simulink model "WithLoad_Simple"  (R2017b)
settings: Solver=ode3  StartTime=0.0  StopTime=10  FixedStep=0.005  RelTol=1e-3  EnableMultiTasking=on
libraries: mblibv1 x61
(part 1 of 3)
settings Model: MAModelExclusionFileProxy=C:\Users\Jiao\Documents\MATLAB\ARNSC_identify_DYN_para\WithLoad_Simple_exclusions.xml  Creator=Robot_One  LastModifiedBy=Chunting
settings DataIOCC: LimitDataPoints=on  SaveFormat=Array
settings OptimizationCC: ExpressionDepthLimit=2147483647  LifeSpan=inf
settings DebuggingCC: UnderspecifiedInitializationDetection=Classic  MergeDetectMultiDrivingBlocksExec=none  SolverPrmCheckMsg=warning  StateNameClashWarn=warning  SFUnexpectedBacktrackingDiag=warning  SFNoUnconditionalDefaultTransitionDiag=warning  SFExecutionAtInitializationDiag=none
settings HardwareCC: ProdBitPerPointer=32  ProdBitPerSizeT=32  ProdBitPerPtrDiffT=32  ProdLargestAtomicFloat=None  ProdIntDivRoundTo=Undefined  ProdEndianess=Unspecified  ProdWordSize=32  ProdHWDeviceType=32-bit Generic
settings ModelReferenceCC: PropagateSignalLabelsOutOfModel=off
settings CodeAppCC: StateflowObjectComments=on
settings GRTTargetCC: TargetLangStandard=C89/C90 (ANSI)  GeneratePreprocessorConditionals=Disable all
settings ConfigComp: CovMetricSettings=dw  CovHtmlReporting=on  CovSaveCumulativeToWorkspaceVar=on  CovSaveSingleToWorkspaceVar=on  CovExternalEMLEnable=off
settings SimscapeCC: SimscapeNormalizeSystem=off
settings SimMechanicsCC: VisDuringSimulation=on  HighlightModel=off  AutoFitVis=GROWTOFIT  LastVizWinPosition=[1 41 1366 626]  CamPosition=[-3.72812;3.39912;13.5529;]  CamTarget=[1.16146;-0.0373873;0.128842;]  CamUpVector=[0.163931;0.968356;-0.188185;]  CamHeight=2.35418  VisBackgroundColor=[0;0;0;]  DefaultBodyColor=[1;0;0;]
settings ConfigurationSet: Description=SimMechanics 2G

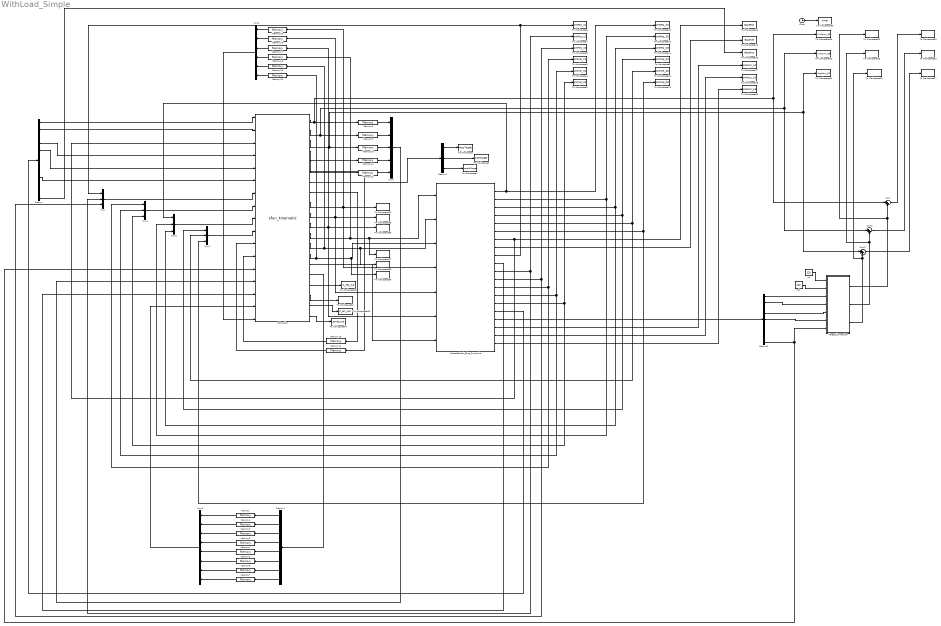
== system WithLoad_Simple ==
  Clock : Clock
  Demux : Demux  Outputs=12
  Demux1 : Demux  Outputs=8
  Demux2 : Demux  Outputs=9
  Demux4 : Demux  Outputs=3
  Memory{,1..10,12..20} (20 alike) : Memory
  Memory11 : Memory  InitialCondition=0.087
  Mux{,1,3..4} (4 alike) : Mux  Inputs=3
  Mux2 : Mux  Inputs=6
  Mux6 : Mux  Inputs=8
  Mux7 : Mux  Inputs=5
  S-Function : S-Function  FunctionName=sfun_kinematic  SFunctionDeploymentMode=off  EnableBusSupport=off
  SpaceRobotic_Blue_Dynamics : Subsystem
  Sum : Sum  Inputs=|++
  Sum1 : Sum  Inputs=|++
  Sum2 : Sum  Inputs=|++
  Target_Momentum : MATLAB Function  TreatAsAtomicUnit=on
  To Workspace : ToWorkspace  VariableName=MassTarget  SaveFormat=Timeseries  SampleTime=-1
  To Workspace1 : ToWorkspace  VariableName=InertiaTarget  SaveFormat=Timeseries  SampleTime=-1
  To Workspace10 : ToWorkspace  VariableName=JointVel_D2  SaveFormat=Timeseries  SampleTime=-1
  To Workspace11 : ToWorkspace  VariableName=JointVel_D3  SaveFormat=Timeseries  SampleTime=-1
  To Workspace12 : ToWorkspace  VariableName=JointPos_D1  SaveFormat=Timeseries  SampleTime=-1
  To Workspace13 : ToWorkspace  VariableName=JointPos_D2  SaveFormat=Timeseries  SampleTime=-1
  To Workspace14 : ToWorkspace  VariableName=JointPos_D3  SaveFormat=Timeseries  SampleTime=-1
  To Workspace15 : ToWorkspace  VariableName=BaseVel  SaveFormat=Timeseries  SampleTime=-1
  To Workspace16 : ToWorkspace  VariableName=BasePos  SaveFormat=Timeseries  SampleTime=-1
  To Workspace17 : ToWorkspace  VariableName=JointAcc_U1  SaveFormat=Timeseries  SampleTime=-1
  To Workspace18 : ToWorkspace  VariableName=JointAcc_U2  SaveFormat=Timeseries  SampleTime=-1
  To Workspace19 : ToWorkspace  VariableName=LinMomX_SR  SaveFormat=Timeseries  SampleTime=-1
  To Workspace2 : ToWorkspace  VariableName=CoMTarget  SaveFormat=Timeseries  SampleTime=-1
  To Workspace20 : ToWorkspace  VariableName=LinMomY_SR  SaveFormat=Timeseries  SampleTime=-1
  To Workspace21 : ToWorkspace  VariableName=AngMom_SR  SaveFormat=Timeseries  SampleTime=-1
  To Workspace22 : ToWorkspace  VariableName=LinMomX_Target  SaveFormat=Timeseries  SampleTime=-1
  To Workspace23 : ToWorkspace  VariableName=LinMomY_Target  SaveFormat=Timeseries  SampleTime=-1
  To Workspace24 : ToWorkspace  VariableName=AngMom_Target  SaveFormat=Timeseries  SampleTime=-1
  To Workspace25 : ToWorkspace  VariableName=LinMomX_Sum  SaveFormat=Timeseries  SampleTime=-1
  To Workspace26 : ToWorkspace  VariableName=LinMomY_Sum  SaveFormat=Timeseries  SampleTime=-1
  To Workspace27 : ToWorkspace  VariableName=AngMom_Sum  SaveFormat=Timeseries  SampleTime=-1
  To Workspace28 : ToWorkspace  VariableName=JointAcc_U3  SaveFormat=Timeseries  SampleTime=-1
  To Workspace29 : ToWorkspace  VariableName=BaseAcc  SaveFormat=Timeseries  SampleTime=-1
  To Workspace3 : ToWorkspace  VariableName=JointVel_U1  SaveFormat=Timeseries  SampleTime=-1
  To Workspace30 : ToWorkspace  VariableName=timer  SaveFormat=Timeseries  SampleTime=-1
  To Workspace31 : ToWorkspace  VariableName=C_eta_out  SaveFormat=Timeseries  SampleTime=-1
  To Workspace32 : ToWorkspace  VariableName=Angle_Err_out  SaveFormat=Timeseries  SampleTime=-1
  To Workspace33 : ToWorkspace  VariableName=K_Err_out  SaveFormat=Timeseries  SampleTime=-1
  To Workspace34 : ToWorkspace  VariableName=JointTorque_U1  SaveFormat=Timeseries  SampleTime=-1
  To Workspace35 : ToWorkspace  VariableName=JointTorque_U2  SaveFormat=Timeseries  SampleTime=-1
  To Workspace36 : ToWorkspace  VariableName=JointTorque_U3  SaveFormat=Timeseries  SampleTime=-1
  To Workspace37 : ToWorkspace  VariableName=JointTorque_D1  SaveFormat=Timeseries  SampleTime=-1
  To Workspace38 : ToWorkspace  VariableName=JointTorque_D2  SaveFormat=Timeseries  SampleTime=-1
  To Workspace39 : ToWorkspace  VariableName=JointTorque_D3  SaveFormat=Timeseries  SampleTime=-1
  To Workspace4 : ToWorkspace  VariableName=JointVel_U2  SaveFormat=Timeseries  SampleTime=-1
  To Workspace40 : ToWorkspace  VariableName=Lamda_out  SaveFormat=Timeseries  SampleTime=-1
  To Workspace5 : ToWorkspace  VariableName=JointVel_U3  SaveFormat=Timeseries  SampleTime=-1
  To Workspace6 : ToWorkspace  VariableName=JointPos_U1  SaveFormat=Timeseries  SampleTime=-1
  To Workspace7 : ToWorkspace  VariableName=JointPos_U2  SaveFormat=Timeseries  SampleTime=-1
  To Workspace8 : ToWorkspace  VariableName=JointPos_U3  SaveFormat=Timeseries  SampleTime=-1
  To Workspace9 : ToWorkspace  VariableName=JointVel_D1  SaveFormat=Timeseries  SampleTime=-1
  mt : Constant  Value=120
  mt1 : Constant  Value=120
  wires:
  S-Function/1 -> Memory8/1, Sum/1, To Workspace19/1  "Base_x_out"
  SpaceRobotic_Blue_Dynamics/7(Base_Ang) -> To Workspace16/1, S-Function/3  "Theta0_in"
  Mux/1 -> S-Function/7  "Theta_U_in"
  Mux1/1 -> S-Function/8  "dTheta_U_in"
  Mux3/1 -> S-Function/9  "Theta_D_in"
  Mux4/1 -> S-Function/10  "dTheta_D_in"
  SpaceRobotic_Blue_Dynamics/11(Link_Ang_U2) -> To Workspace7/1, Mux/2
  SpaceRobotic_Blue_Dynamics/12(Link_Ang_U3) -> To Workspace8/1, Mux/3
  SpaceRobotic_Blue_Dynamics/13(Link_Ang_U1_w) -> To Workspace3/1, Mux1/1
  SpaceRobotic_Blue_Dynamics/14(Link_Ang_U2_w) -> To Workspace4/1, Mux1/2
  SpaceRobotic_Blue_Dynamics/15(Link_Ang_U3_w) -> To Workspace5/1, Mux1/3
  SpaceRobotic_Blue_Dynamics/1(Link_Ang_D1) -> Mux3/1, To Workspace12/1
  SpaceRobotic_Blue_Dynamics/2(Link_Ang_D2) -> To Workspace13/1, Mux3/2
  SpaceRobotic_Blue_Dynamics/3(Link_Ang_D3) -> To Workspace14/1, Mux3/3
  SpaceRobotic_Blue_Dynamics/4(Link_Ang_D1_w) -> To Workspace9/1, Mux4/1
  SpaceRobotic_Blue_Dynamics/5(Link_Ang_D2_w) -> To Workspace10/1, Mux4/2
  SpaceRobotic_Blue_Dynamics/6(Link_Ang_D3_w) -> To Workspace11/1, Mux4/3
  S-Function/2 -> Sum1/1, To Workspace20/1, Memory9/1  "Base_y_out"
  S-Function/3 -> To Workspace21/1, Sum2/1, Memory10/1  "L_out"
  Demux/1 -> S-Function/1  "Base_x_in"
  Demux/2 -> S-Function/2  "Base_y_in"
  SpaceRobotic_Blue_Dynamics/16(r_0) -> Demux/1
  Demux/4 -> S-Function/4  "Base_vx_in"
  Demux/5 -> S-Function/5  "Base_vy_in"
  Demux/9 -> S-Function/6  "dTheta0_in"
  S-Function/14 -> Memory20/1, To Workspace39/1, SpaceRobotic_Blue_Dynamics/3(Link_Actuator_D3)  "Tau3_D"
  S-Function/13 -> Memory19/1, To Workspace38/1, SpaceRobotic_Blue_Dynamics/2(Link_Actuator_D2)  "Tau2_D"
  S-Function/12 -> Memory18/1, To Workspace37/1, SpaceRobotic_Blue_Dynamics/1(Link_Actuator_D1)  "Tau1_D"
  S-Function/11 -> SpaceRobotic_Blue_Dynamics/6(Link_Actuator_U3), Memory17/1, To Workspace36/1  "Tau3_U"
  S-Function/10 -> Memory16/1, To Workspace35/1, SpaceRobotic_Blue_Dynamics/5(Link_Actuator_U2)  "Tau2_U"
  S-Function/9 -> Memory15/1, To Workspace34/1, SpaceRobotic_Blue_Dynamics/4(Link_Actuator_U1)  "Tau1_U"
  S-Function/15 -> SpaceRobotic_Blue_Dynamics/7(Counter)  "Counter"
  S-Function/16 -> Demux1/1  "Iteration_out"
  Mux6/1 -> S-Function/16
  Demux1/1 -> Memory/1
  Demux1/2 -> Memory1/1
  Demux1/3 -> Memory2/1
  Demux1/4 -> Memory3/1
  Demux1/5 -> Memory4/1
  Demux1/6 -> Memory5/1
  Demux1/7 -> Memory6/1
  Demux1/8 -> Memory7/1
  Memory/1 -> Mux6/1
  Memory1/1 -> Mux6/2
  Memory2/1 -> Mux6/3
  Memory3/1 -> Mux6/4
  Memory4/1 -> Mux6/5
  Memory5/1 -> Mux6/6
  Memory6/1 -> Mux6/7
  Memory7/1 -> Mux6/8
  SpaceRobotic_Blue_Dynamics/8(Base_Ang_w) -> To Workspace15/1
  SpaceRobotic_Blue_Dynamics/17(Target_p_v_w) -> Demux2/1
  mt/1 -> Target_Momentum/1(mt)
  mt1/1 -> Target_Momentum/2(It)
  Target_Momentum/1(Px) -> Sum/2, To Workspace22/1
  Target_Momentum/2(Py) -> Sum1/2, To Workspace23/1
  Target_Momentum/3(L) -> Sum2/2, To Workspace24/1
  Demux2/1 -> Target_Momentum/3(rx)
  Demux2/2 -> Target_Momentum/4(ry)
  Demux2/4 -> Target_Momentum/5(vx)
  Demux2/5 -> Target_Momentum/6(vy)
  Demux2/9 -> S-Function/13, Target_Momentum/7(wz)
  Sum/1 -> To Workspace25/1
  Sum1/1 -> To Workspace26/1
  Sum2/1 -> To Workspace27/1
  SpaceRobotic_Blue_Dynamics/10(EndEffect_U_ve_w) -> S-Function/15  "EndEffect_U_ve_w_in"
  Mux7/1 -> S-Function/14
  Memory8/1 -> Mux7/1
  Memory9/1 -> Mux7/2
  Memory10/1 -> Mux7/3
  S-Function/4 -> Memory11/1  "dTheta_Ue_out"
  Memory11/1 -> Mux7/4
  Memory12/1 -> Mux7/5
  S-Function/5 -> Memory12/1  "dTheta_U_out"
  Demux4/1 -> To Workspace/1
  Demux4/2 -> To Workspace2/1
  Demux4/3 -> To Workspace1/1
  S-Function/7 -> Demux4/1  "id_Results_out"
  S-Function/8 -> Memory13/1  "ddTheta_D_out"
  Memory13/1 -> S-Function/12  "Link_CG_ddR_U_in"
  S-Function/6 -> Memory14/1  "Pe_The_out"
  Memory14/1 -> S-Function/11  "Pe_The_t_1_in"
  SpaceRobotic_Blue_Dynamics/18(Link_Ang_U1_a) -> To Workspace17/1
  SpaceRobotic_Blue_Dynamics/19(Link_Ang_U2_a) -> To Workspace18/1
  SpaceRobotic_Blue_Dynamics/20(Link_Ang_U3_a) -> To Workspace28/1
  Demux/12 -> To Workspace29/1
  Clock/1 -> To Workspace30/1
  S-Function/17 -> To Workspace31/1
  S-Function/18 -> To Workspace32/1
  S-Function/19 -> To Workspace33/1
  SpaceRobotic_Blue_Dynamics/9(Link_Ang_U1) -> To Workspace6/1, Mux/1
  Memory15/1 -> Mux2/1
  Memory16/1 -> Mux2/2
  Memory17/1 -> Mux2/3
  Memory18/1 -> Mux2/4
  Memory19/1 -> Mux2/5
  Memory20/1 -> Mux2/6
  Mux2/1 -> S-Function/17
  S-Function/20 -> To Workspace40/1
